simulink model "modelloSatelliteParamNoti"  (R2025b)
settings: Solver=VariableStepAuto  StartTime=0.0  StopTime=3  RelTol=1e-3
values from neighbouring files (symbols this model uses):
  I = [13470; 20450; 27200]    [main.m]
  K = diag([20 20 20])    [main.m]
settings Model: Creator=Armando  LastModifiedBy=Armando

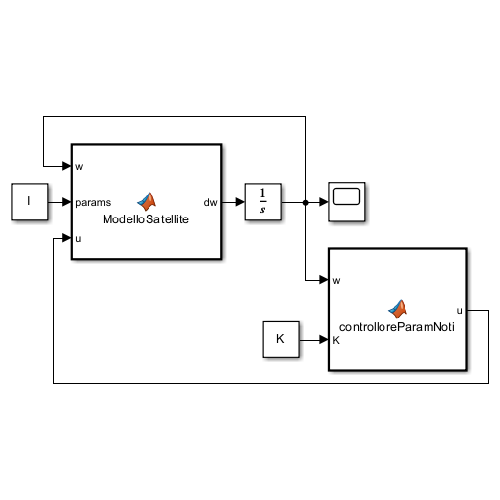
[thumbnail: Simulink's stored preview of the top-level diagram]
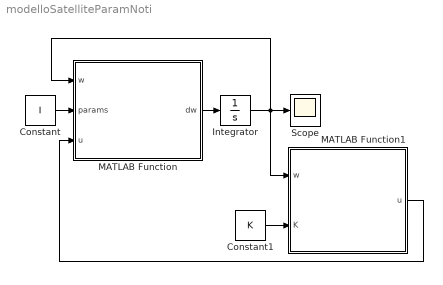
== system modelloSatelliteParamNoti ==
  Constant : Constant  Value=I
  Constant1 : Constant  Value=K
  Integrator : Integrator  InitialCondition=[1;1;1]
  MATLAB Function : MATLAB Function  TreatAsAtomicUnit=on
  MATLAB Function1 : MATLAB Function  TreatAsAtomicUnit=on
  Scope : Scope
      settings: ActiveDisplayYMinimum=-0.125  ActiveDisplayYMaximum=1.125
  wires:
  Constant/1 -> MATLAB Function/2(params)
  MATLAB Function/1(dw) -> Integrator/1
  Integrator/1 -> MATLAB Function1/1(w), Scope/1, MATLAB Function/1(w)
  Constant1/1 -> MATLAB Function1/2(K)
  MATLAB Function1/1(u) -> MATLAB Function/3(u)

== matlab function modelloSatelliteParamNoti/MATLAB Function ==
  data: w input; params input; u input; dw output
function dw = ModelloSatellite(w,params,u)
    c = [(params(2) - params(3))/params(1)*w(2)*w(3);
         ( params(3)- params(1))/params(2)*w(3)*w(1);
          (params(1) - params(2))/params(3)*w(1)*w(2)];
    
    dw = c + (u/params(:));

== matlab function modelloSatelliteParamNoti/MATLAB Function1 ==
  data: w input; u output; K input
function u = controlloreParamNoti(w,K)
    u = -K*w;
